simulink model "PC_Quadcopter_Simulation_Alchemist"  (R2023b)
settings: Solver=ode4  StartTime=0  StopTime=Tf  FixedStep=Ts  MaxStep=0.06  RelTol=1e-3  EnableMultiTasking=on
model workspace (MAT data in the model file):
  Sig : Simulink.Signal (value not decoded)
values from neighbouring files (symbols this model uses):
  den_Pphi = conv(den_Qphi, num_Gphi)    [PC_Quadcopter_Alchemist_woDOBC.m]    (also in workingOcto.m)
  den_Ppsi = conv(den_Qpsi, num_Gpsi)    [PC_Quadcopter_Alchemist_woDOBC.m]    (also in workingOcto.m)
  den_Ptheta = conv(den_Qtheta, num_Gtheta)    [PC_Quadcopter_Alchemist_woDOBC.m]    (also in workingOcto.m)
  den_Px = conv(den_Qx, num_Gx)    [PC_Quadcopter_Alchemist_woDOBC.m]    (also in workingOcto.m)
  den_Py = conv(den_Qy, num_Gy)    [PC_Quadcopter_Alchemist_woDOBC.m]    (also in workingOcto.m)
  den_Pz = conv(den_Qz, num_Gz)    [PC_Quadcopter_Alchemist_woDOBC.m]    (also in workingOcto.m)
  Dist_Amp_phi = 0    [PC_Quadcopter_Alchemist_woDOBC.m]    (also in workingOcto.m)
  Dist_Amp_psi = 0    [PC_Quadcopter_Alchemist_woDOBC.m]    (also in workingOcto.m)
  Dist_Amp_theta = 0    [PC_Quadcopter_Alchemist_woDOBC.m]    (also in workingOcto.m)
  Dist_Amp_x = 0    [PC_Quadcopter_Alchemist_woDOBC.m]    (also in workingOcto.m)
  Dist_Amp_y = 0    [PC_Quadcopter_Alchemist_woDOBC.m]    (also in workingOcto.m)
  Dist_Amp_z = 0    [PC_Quadcopter_Alchemist_woDOBC.m]    (also in workingOcto.m)
  Dist_Freq_phi = 0    [PC_Quadcopter_Alchemist_woDOBC.m]    (also in workingOcto.m)
  Dist_Freq_psi = 0    [PC_Quadcopter_Alchemist_woDOBC.m]    (also in workingOcto.m)
  Dist_Freq_theta = 0    [PC_Quadcopter_Alchemist_woDOBC.m]    (also in workingOcto.m)
  Dist_Freq_x = 0    [PC_Quadcopter_Alchemist_woDOBC.m]    (also in workingOcto.m)
  Dist_Freq_y = 0    [PC_Quadcopter_Alchemist_woDOBC.m]    (also in workingOcto.m)
  Dist_Freq_z = 0    [PC_Quadcopter_Alchemist_woDOBC.m]    (also in workingOcto.m)
  Dist_mean_phi = 0    [PC_Quadcopter_Alchemist_woDOBC.m]    (also in workingOcto.m)
  Dist_mean_psi = 0    [PC_Quadcopter_Alchemist_woDOBC.m]    (also in workingOcto.m)
  Dist_mean_theta = 0    [PC_Quadcopter_Alchemist_woDOBC.m]    (also in workingOcto.m)
  Dist_mean_x = 0    [PC_Quadcopter_Alchemist_woDOBC.m]    (also in workingOcto.m)
  Dist_mean_y = 0    [PC_Quadcopter_Alchemist_woDOBC.m]    (also in workingOcto.m)
  Dist_mean_z = 0    [PC_Quadcopter_Alchemist_woDOBC.m]    (also in workingOcto.m)
  Dist_Var_phi = 0    [PC_Quadcopter_Alchemist_woDOBC.m]    (also in workingOcto.m)
  Dist_Var_psi = 0    [PC_Quadcopter_Alchemist_woDOBC.m]    (also in workingOcto.m)
  Dist_Var_theta = 0    [PC_Quadcopter_Alchemist_woDOBC.m]    (also in workingOcto.m)
  Dist_Var_x = 0    [PC_Quadcopter_Alchemist_woDOBC.m]    (also in workingOcto.m)
  Dist_Var_y = 0    [PC_Quadcopter_Alchemist_woDOBC.m]    (also in workingOcto.m)
  Dist_Var_z = 0    [PC_Quadcopter_Alchemist_woDOBC.m]    (also in workingOcto.m)
  DISTURBANCE = 0    [PC_Quadcopter_Alchemist_woDOBC.m]    (also in workingOcto.m)
  DOBC_phi = 0    [PC_Quadcopter_Alchemist_woDOBC.m]    (also in workingOcto.m)
  DOBC_psi = 0    [PC_Quadcopter_Alchemist_woDOBC.m]    (also in workingOcto.m)
  DOBC_theta = 0    [PC_Quadcopter_Alchemist_woDOBC.m]    (also in workingOcto.m)
  DOBC_x = 0    [PC_Quadcopter_Alchemist_woDOBC.m]    (also in workingOcto.m)
  DOBC_y = 0    [PC_Quadcopter_Alchemist_woDOBC.m]    (also in workingOcto.m)
  DOBC_z = 0    [PC_Quadcopter_Alchemist_woDOBC.m]    (also in workingOcto.m)
  GO = (sqrt((m*g)/(8*ct))-b)/cr    [PC_Quadcopter_Alchemist_woDOBC.m]    (also in workingOcto.m)
  IC =     [Hover_1m.mat]    (also in quadcopterDynamicsSFunction_Alchemist.m = block.DialogPrm(2).Data)
  INPUT_MODE_PHI = 0    [PC_Quadcopter_Alchemist_woDOBC.m]    (also in workingOcto.m)
  INPUT_MODE_THETA = 0    [PC_Quadcopter_Alchemist_woDOBC.m]    (also in workingOcto.m)
  INPUT_MODE_U = 0    [PC_Quadcopter_Alchemist_woDOBC.m]    (also in workingOcto.m)
  INPUT_MODE_V = 0    [PC_Quadcopter_Alchemist_woDOBC.m]    (also in workingOcto.m)
  Kd_phi = 2*Zc_phi*Wc_phi*Jx/Kphi    [PC_Quadcopter_Alchemist_woDOBC.m]    (also in workingOcto.m)
  Kd_psi = 2*Zc_psi*Wc_psi*Jz/Kpsi    [PC_Quadcopter_Alchemist_woDOBC.m]    (also in workingOcto.m)
  Kd_theta = 2*Zc_theta*Wc_theta*Jy/Ktheta    [PC_Quadcopter_Alchemist_woDOBC.m]    (also in workingOcto.m)
  Kd_u = Kp_u/50    [PC_Quadcopter_Alchemist_woDOBC.m]    (also in workingOcto.m)
  Kd_v = Kp_v/70    [PC_Quadcopter_Alchemist_woDOBC.m]    (also in workingOcto.m)
  Kd_x = Kp_x/5    (= 0.0710753921948)    [PC_Quadcopter_Alchemist_woDOBC.m]    (also in workingOcto.m = Kp_x/5)
  Kd_y = Kp_y/5    (= 0.014215078439)    [PC_Quadcopter_Alchemist_woDOBC.m]    (also in workingOcto.m = Kp_y/5)
  Kd_z = 2*Zc_z*Wc_z*m/Kz    [PC_Quadcopter_Alchemist_woDOBC.m]    (also in workingOcto.m = Kp_z/10)
  Ki_phi = Kp_phi/10    [PC_Quadcopter_Alchemist_woDOBC.m]    (also in workingOcto.m)
  Ki_psi = Kp_psi/20    [PC_Quadcopter_Alchemist_woDOBC.m]    (also in workingOcto.m)
  Ki_theta = Kp_theta/10    [PC_Quadcopter_Alchemist_woDOBC.m]    (also in workingOcto.m)
  Ki_u = Wc_u^2/g * 0.7    [PC_Quadcopter_Alchemist_woDOBC.m]    (also in workingOcto.m)
  Ki_v = Wc_v^2/g * 0.7    [PC_Quadcopter_Alchemist_woDOBC.m]    (also in workingOcto.m)
  Ki_x = Wc_x^2 * 0.7    (= 0.0442158277169)    [PC_Quadcopter_Alchemist_woDOBC.m]    (also in workingOcto.m = Wc_x^2 * 0.7)
  Ki_y = Wc_y^2 * 0.7    (= 0.00176863310868)    [PC_Quadcopter_Alchemist_woDOBC.m]    (also in workingOcto.m = Wc_y^2 * 0.7)
  Ki_z = 0    [PC_Quadcopter_Alchemist_woDOBC.m]    (also in workingOcto.m = Wc_z^2)
  Kp_phi = Wc_phi^2*Jx/Kphi    [PC_Quadcopter_Alchemist_woDOBC.m]    (also in workingOcto.m)
  Kp_psi = Wc_psi^2*Jz/Kpsi    [PC_Quadcopter_Alchemist_woDOBC.m]    (also in workingOcto.m)
  Kp_theta = Wc_theta^2*Jy/Ktheta    [PC_Quadcopter_Alchemist_woDOBC.m]    (also in workingOcto.m)
  Kp_u = 2*Zc_u*Wc_u/g    [PC_Quadcopter_Alchemist_woDOBC.m]    (also in workingOcto.m)
  Kp_v = 2*Zc_v*Wc_v/g    [PC_Quadcopter_Alchemist_woDOBC.m]    (also in workingOcto.m)
  Kp_x = 2*Wc_x*Zc_x    (= 0.355376960974)    [PC_Quadcopter_Alchemist_woDOBC.m]    (also in workingOcto.m = 2*Wc_x*Zc_x)
  Kp_y = 2*Wc_y*Zc_y    (= 0.0710753921948)    [PC_Quadcopter_Alchemist_woDOBC.m]    (also in workingOcto.m = 2*Wc_y*Zc_y)
  Kp_z = Wc_z^2*Jz/Kz    [PC_Quadcopter_Alchemist_woDOBC.m]    (also in workingOcto.m = 2*Wc_z*Zc_z)
  NOISE = 0    [PC_Quadcopter_Alchemist_woDOBC.m]    (also in workingOcto.m)
  num_Pphi = conv(num_Qphi, den_Gphi)    [PC_Quadcopter_Alchemist_woDOBC.m]    (also in workingOcto.m)
  num_Ppsi = conv(num_Qpsi, den_Gpsi)    [PC_Quadcopter_Alchemist_woDOBC.m]    (also in workingOcto.m)
  num_Ptheta = conv(num_Qtheta, den_Gtheta)    [PC_Quadcopter_Alchemist_woDOBC.m]    (also in workingOcto.m)
  num_Px = conv(num_Qx, den_Gx)    [PC_Quadcopter_Alchemist_woDOBC.m]    (also in workingOcto.m)
  num_Py = conv(num_Qy, den_Gy)    [PC_Quadcopter_Alchemist_woDOBC.m]    (also in workingOcto.m)
  num_Pz = conv(num_Qz, den_Gz)    [PC_Quadcopter_Alchemist_woDOBC.m]    (also in workingOcto.m)
  Phid = deg2rad(1)    [PC_Quadcopter_Alchemist_woDOBC.m]    (also in workingOcto.m = deg2rad(5))
  start_time = 5    [PC_Quadcopter_Alchemist_woDOBC.m]    (also in workingOcto.m = 1)
  step_0_ramp_1 = 0    [PC_Quadcopter_Alchemist_woDOBC.m]    (also in workingOcto.m)
  Thetad = deg2rad(1)    [PC_Quadcopter_Alchemist_woDOBC.m]    (also in workingOcto.m = deg2rad(0))
  Ts = 0.01    [PC_Quadcopter_Alchemist_woDOBC.m]    (also in workingOcto.m)
  Ud = 0    [PC_Quadcopter_Alchemist_woDOBC.m]    (also in workingOcto.m)
  Var_phi = 0.005^2    (= 2.5e-05)    [PC_Quadcopter_Alchemist_woDOBC.m]    (also in workingOcto.m)
  Var_psi = 0.005^2    (= 2.5e-05)    [PC_Quadcopter_Alchemist_woDOBC.m]    (also in workingOcto.m)
  Var_theta = 0.005^2    (= 2.5e-05)    [PC_Quadcopter_Alchemist_woDOBC.m]    (also in workingOcto.m)
  Var_u = 0.01^2    (= 0.0001)    [PC_Quadcopter_Alchemist_woDOBC.m]    (also in workingOcto.m)
  Var_v = 0.01^2    (= 0.0001)    [PC_Quadcopter_Alchemist_woDOBC.m]    (also in workingOcto.m)
  Var_w = 0.01^2    (= 0.0001)    [PC_Quadcopter_Alchemist_woDOBC.m]    (also in workingOcto.m)
  Var_x = 0.01^2    (= 0.0001)    [PC_Quadcopter_Alchemist_woDOBC.m]    (also in workingOcto.m)
  Var_y = 0.01^2    (= 0.0001)    [PC_Quadcopter_Alchemist_woDOBC.m]    (also in workingOcto.m)
  Var_z = 0.01^2    (= 0.0001)    [PC_Quadcopter_Alchemist_woDOBC.m]    (also in workingOcto.m)
  Vd = 0    [PC_Quadcopter_Alchemist_woDOBC.m]    (also in workingOcto.m)
  Vz = 0.1    [PC_Quadcopter_Alchemist_woDOBC.m]    (also in workingOcto.m)
  Xd = 0    [PC_Quadcopter_Alchemist_woDOBC.m]    (also in workingOcto.m = 1)
  Yd = 0    [PC_Quadcopter_Alchemist_woDOBC.m]    (also in workingOcto.m = 1)
  Zd = 2    [PC_Quadcopter_Alchemist_woDOBC.m]    (also in workingOcto.m = 1)
undefined symbols (not defined in the file or in its folder): den_Qphi, den_Qpsi, den_Qtheta, den_Qx, den_Qy, den_Qz, num_Qphi, num_Qpsi, num_Qtheta, num_Qx, num_Qy, num_Qz, quadModel
libraries: simulink x10, slpidlib x2, sharedtransform x1, uavutilslib x1
(part 2 of 2)

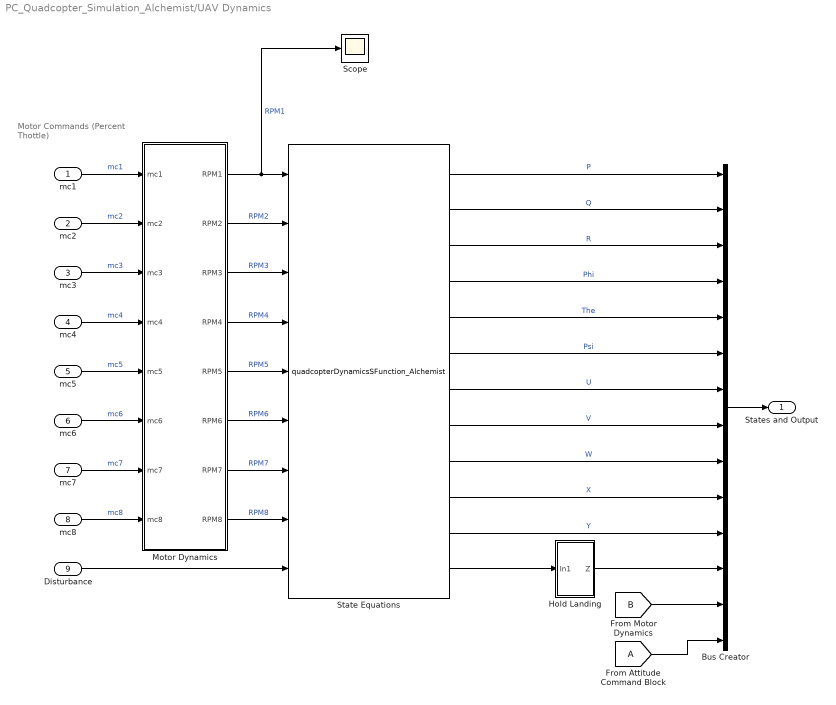
== system PC_Quadcopter_Simulation_Alchemist/UAV Dynamics ==
  note: Motor Commands
      | (Percent Thottle)
  mc1 : Inport
  mc2 : Inport  Port=2
  mc3 : Inport  Port=3
  mc4 : Inport  Port=4
  mc5 : Inport  Port=5
  mc6 : Inport  Port=6
  mc7 : Inport  Port=7
  mc8 : Inport  Port=8
  Disturbance : Inport  Port=9
  Bus Creator : BusCreator  Inputs='P','Q','R','Phi','The','Psi','U','V','W','X','Y','Z','mc and RPM','Attitude_Cmd'
  From Attitude Command Block : From  TagVisibility=global
  Hold Landing : Subsystem
  Motor Dynamics : Subsystem
  Scope : Scope
  State Equations : M-S-Function  FunctionName=quadcopterDynamicsSFunction_Alchemist  Parameters=quadModel, IC
      mask Display:
      | port_label('input', 1, 'RPM1')
      | port_label('input', 2, 'RPM2')
      | port_label('input', 3, 'RPM3')
      | port_label('input', 4, 'RPM4')
      | port_label('input', 5, 'Disturbances')
      | port_label('output', 1, 'P')
      | port_label('output', 2, 'Q')
      | port_label('output', 3, 'R')
      | port_label('output', 4, 'Phi')
      | port_label('output', 5, 'The')
      | port_label('output', 6, 'Psi')
      | port_label('output', 7, 'U')
      | port_label('output', 8, 'V')
      | port_label('output', 9, 'W')
      | port_label('output', 10, 'X')
      | port_label('output', 11, 'Y')
      | port_label('output', 12, 'Z')
  States and Output : Outport  VectorParamsAs1DForOutWhenUnconnected=off
  wires:
  [B] -> Bus Creator/13
  From Attitude Command Block/1 -> Bus Creator/14
  mc2/1 -> Motor Dynamics/2(mc2)  "mc2"
  mc3/1 -> Motor Dynamics/3(mc3)  "mc3"
  mc4/1 -> Motor Dynamics/4(mc4)  "mc4"
  mc1/1 -> Motor Dynamics/1(mc1)  "mc1"
  Motor Dynamics/3(RPM3) -> State Equations/3  "RPM3"
  Motor Dynamics/2(RPM2) -> State Equations/2  "RPM2"
  Bus Creator/1 -> States and Output/1
  State Equations/11 -> Bus Creator/11  "Y"
  State Equations/10 -> Bus Creator/10  "X"
  State Equations/9 -> Bus Creator/9  "W"
  State Equations/8 -> Bus Creator/8  "V"
  State Equations/7 -> Bus Creator/7  "U"
  State Equations/6 -> Bus Creator/6  "Psi"
  State Equations/5 -> Bus Creator/5  "The"
  State Equations/4 -> Bus Creator/4  "Phi"
  State Equations/3 -> Bus Creator/3  "R"
  State Equations/2 -> Bus Creator/2  "Q"
  State Equations/1 -> Bus Creator/1  "P"
  Motor Dynamics/1(RPM1) -> Scope/1, State Equations/1  "RPM1"
  mc5/1 -> Motor Dynamics/5(mc5)  "mc5"
  mc6/1 -> Motor Dynamics/6(mc6)  "mc6"
  State Equations/12 -> Hold Landing/1(In1)
  Hold Landing/1(Z) -> Bus Creator/12
  mc7/1 -> Motor Dynamics/7(mc7)  "mc7"
  mc8/1 -> Motor Dynamics/8(mc8)  "mc8"
  Disturbance/1 -> State Equations/9
  Motor Dynamics/4(RPM4) -> State Equations/4  "RPM4"
  Motor Dynamics/5(RPM5) -> State Equations/5  "RPM5"
  Motor Dynamics/6(RPM6) -> State Equations/6  "RPM6"
  Motor Dynamics/7(RPM7) -> State Equations/7  "RPM7"
  Motor Dynamics/8(RPM8) -> State Equations/8  "RPM8"

== system PC_Quadcopter_Simulation_Alchemist/Attitude & Altitude Controller/Altitude (Z) Control ==
  note: ez
  note: Improve to use rotation matrix and euler angles...
      | maybe with saturation?
  Desired Z : Inport
  Z State : Inport  Port=2
  Bus Selector : BusSelector  OutputSignals=Alt_cmd
  Derivative : Derivative
  Gravity Offset (Level Flight) : Constant  Value=GOffset
  Integrator Limited : Integrator  LimitOutput=on  UpperSaturationLimit=USat  LowerSaturationLimit=LSat
  Kdz : Gain  Gain=Kdz
  Kiz : Gain  Gain=Kiz
  Kpz : Gain  Gain=Kpz
  Sum : Sum  Inputs=|+-
  Sum2 : Sum  Inputs=+++-
  Alt. (Z) Correction : Outport  VectorParamsAs1DForOutWhenUnconnected=off
  wires:
  Derivative/1 -> Kdz/1
  Bus Selector/1 -> Sum/1  "<Alt_cmd>"
  Integrator Limited/1 -> Kiz/1
  Kdz/1 -> Sum2/4  "D Corr"
  Kiz/1 -> Sum2/3  "I Corr"
  Sum/1 -> Kpz/1, Integrator Limited/1  "Error"
  Kpz/1 -> Sum2/2  "P Corr"
  Sum2/1 -> Alt. (Z) Correction/1
  Z State/1 -> Sum/2, Derivative/1
  Desired Z/1 -> Bus Selector/1
  Gravity Offset (Level Flight)/1 -> Sum2/1

== system PC_Quadcopter_Simulation_Alchemist/Attitude & Altitude Controller/DOBC_Phi ==
  In2 : Inport
  Phi : Inport  Port=2
  Gain3 : Gain  Gain=DOBC_phi
  Q(s)*inv(G(s))3 : TransferFcn  Numerator=num_Pphi  Denominator=den_Pphi
  Q(s)3 : TransferFcn  Numerator=num_Qphi  Denominator=den_Qphi
  Sum6 : Sum  Inputs=|+-
  Sum9 : Sum  Inputs=+|-
  Roll (Phi) Correction : Outport
  wires:
  Sum9/1 -> Gain3/1
  Q(s)3/1 -> Sum9/2
  Sum6/1 -> Roll (Phi) Correction/1, Q(s)3/1
  In2/1 -> Sum6/1
  Q(s)*inv(G(s))3/1 -> Sum9/1
  Gain3/1 -> Sum6/2
  Phi/1 -> Q(s)*inv(G(s))3/1

== system PC_Quadcopter_Simulation_Alchemist/Attitude & Altitude Controller/DOBC_Psi ==
  In2 : Inport
  Psi : Inport  Port=2
  Gain1 : Gain  Gain=DOBC_psi
  Q(s)*inv(G(s))1 : TransferFcn  Numerator=num_Ppsi  Denominator=den_Ppsi
  Q(s)1 : TransferFcn  Numerator=num_Qpsi  Denominator=den_Qpsi
  Sum4 : Sum  Inputs=|+-
  Sum7 : Sum  Inputs=+|-
  Yaw (Psi) Correction : Outport
  wires:
  Sum7/1 -> Gain1/1
  Psi/1 -> Q(s)*inv(G(s))1/1
  Sum4/1 -> Yaw (Psi) Correction/1, Q(s)1/1
  Q(s)1/1 -> Sum7/2
  Q(s)*inv(G(s))1/1 -> Sum7/1
  Gain1/1 -> Sum4/2
  In2/1 -> Sum4/1

== system PC_Quadcopter_Simulation_Alchemist/Attitude & Altitude Controller/DOBC_Theta ==
  In2 : Inport
  Theta : Inport  Port=2
  Gain2 : Gain  Gain=DOBC_theta
  Q(s)*inv(G(s))2 : TransferFcn  Numerator=num_Ptheta  Denominator=den_Ptheta
  Q(s)2 : TransferFcn  Numerator=num_Qtheta  Denominator=den_Qtheta
  Sum5 : Sum  Inputs=|+-
  Sum8 : Sum  Inputs=+|-
  Pitch (Theta) Correction : Outport
  wires:
  Gain2/1 -> Sum5/2
  Sum5/1 -> Pitch (Theta) Correction/1, Q(s)2/1
  Sum8/1 -> Gain2/1
  Q(s)*inv(G(s))2/1 -> Sum8/1
  In2/1 -> Sum5/1
  Q(s)2/1 -> Sum8/2
  Theta/1 -> Q(s)*inv(G(s))2/1

== system PC_Quadcopter_Simulation_Alchemist/Attitude & Altitude Controller/DOBC_Z ==
  In1 : Inport
  Z : Inport  Port=2
  Gain : Gain  Gain=DOBC_z
  Q(s) : TransferFcn  Numerator=num_Qz  Denominator=den_Qz
  Q(s)*inv(G(s)) : TransferFcn  Numerator=num_Pz  Denominator=den_Pz
  Sum : Sum  Inputs=+|-
  Sum1 : Sum  Inputs=|+-
  Out1 : Outport
  wires:
  Sum/1 -> Gain/1
  Sum1/1 -> Out1/1, Q(s)/1
  In1/1 -> Sum1/1
  Gain/1 -> Sum1/2
  Q(s)*inv(G(s))/1 -> Sum/1
  Q(s)/1 -> Sum/2
  Z/1 -> Q(s)*inv(G(s))/1

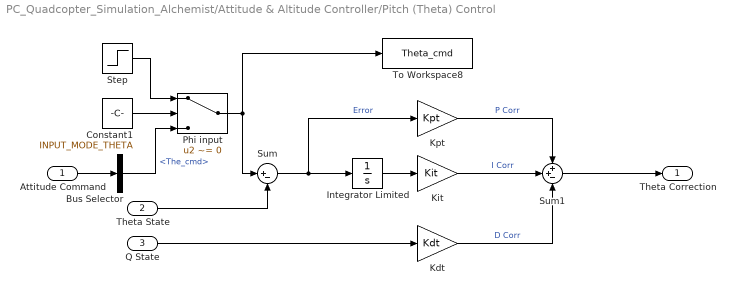
== system PC_Quadcopter_Simulation_Alchemist/Attitude & Altitude Controller/Pitch (Theta) Control ==
  Attitude Command : Inport
  Theta State : Inport  Port=2
  Q State : Inport  Port=3
  Bus Selector : BusSelector  OutputSignals=The_cmd
  Constant1 : Constant  Value=INPUT_MODE_THETA
  Integrator Limited : Integrator  LimitOutput=on  UpperSaturationLimit=USat  LowerSaturationLimit=LSat
  Kdt : Gain  Gain=Kdt
  Kit : Gain  Gain=Kit
  Kpt : Gain  Gain=Kpt
  Phi input : Switch  Criteria=u2 ~= 0  SaturateOnIntegerOverflow=off  InputSameDT=off
  Step : Step  Time=start_time  After=Thetad  SampleTime=0
  Sum : Sum  Inputs=|+-
  Sum1 : Sum  Inputs=++-
  To Workspace8 : ToWorkspace  VariableName=Theta_cmd  SampleTime=-1
      settings: Save2DSignal=2-D array (concatenate along first dimension)
  Theta Correction : Outport  VectorParamsAs1DForOutWhenUnconnected=off
  wires:
  Q State/1 -> Kdt/1
  Bus Selector/1 -> Phi input/3  "<The_cmd>"
  Integrator Limited/1 -> Kit/1
  Kit/1 -> Sum1/2  "I Corr"
  Kdt/1 -> Sum1/3  "D Corr"
  Kpt/1 -> Sum1/1  "P Corr"
  Sum1/1 -> Theta Correction/1
  Theta State/1 -> Sum/2
  Attitude Command/1 -> Bus Selector/1
  Sum/1 -> Kpt/1, Integrator Limited/1  "Error"
  Phi input/1 -> Sum/1, To Workspace8/1
  Step/1 -> Phi input/1
  Constant1/1 -> Phi input/2

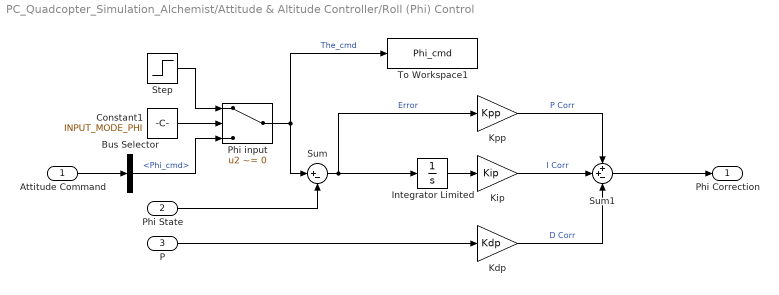
== system PC_Quadcopter_Simulation_Alchemist/Attitude & Altitude Controller/Roll (Phi) Control  ==
  "Attitude Command " : Inport
  Phi State : Inport  Port=2
  P : Inport  Port=3
  Bus Selector : BusSelector  OutputSignals=Phi_cmd
  Constant1 : Constant  Value=INPUT_MODE_PHI
  Integrator Limited : Integrator  LimitOutput=on  UpperSaturationLimit=USat  LowerSaturationLimit=LSat
  Kdp : Gain  Gain=Kdp
  Kip : Gain  Gain=Kip
  Kpp : Gain  Gain=Kpp
  Phi input : Switch  Criteria=u2 ~= 0  SaturateOnIntegerOverflow=off  InputSameDT=off
  Step : Step  Time=start_time  After=Phid  SampleTime=0
  Sum : Sum  Inputs=|+-
  Sum1 : Sum  Inputs=++-
  To Workspace1 : ToWorkspace  VariableName=Phi_cmd  SampleTime=-1
      settings: Save2DSignal=2-D array (concatenate along first dimension)
  Phi Correction : Outport  VectorParamsAs1DForOutWhenUnconnected=off
  wires:
  P/1 -> Kdp/1
  Bus Selector/1 -> Phi input/3  "<Phi_cmd>"
  "Attitude Command "/1 -> Bus Selector/1
  Integrator Limited/1 -> Kip/1
  Kip/1 -> Sum1/2  "I Corr"
  Kdp/1 -> Sum1/3  "D Corr"
  Kpp/1 -> Sum1/1  "P Corr"
  Sum1/1 -> Phi Correction/1
  Phi State/1 -> Sum/2
  Sum/1 -> Kpp/1, Integrator Limited/1  "Error"
  Step/1 -> Phi input/1
  Constant1/1 -> Phi input/2
  Phi input/1 -> To Workspace1/1, Sum/1  "The_cmd"

== system PC_Quadcopter_Simulation_Alchemist/Attitude & Altitude Controller/Yaw (Psi) Control ==
  Attitude Command : Inport
  Psi State : Inport  Port=2
  R State : Inport  Port=3
  Bus Selector : BusSelector  OutputSignals=Psi_cmd
  Integrator Limited : Integrator  LimitOutput=on  UpperSaturationLimit=USat  LowerSaturationLimit=LSat
  Kds : Gain  Gain=Kds
  Kit : Gain  Gain=Kis
  Kps : Gain  Gain=Kps
  Sum : Sum  Inputs=|+-
  Sum1 : Sum  Inputs=++-
  To Workspace3 : ToWorkspace  VariableName=Psi_cmd  SampleTime=-1
      settings: Save2DSignal=2-D array (concatenate along first dimension)
  Psi Correction : Outport  VectorParamsAs1DForOutWhenUnconnected=off
  wires:
  R State/1 -> Kds/1
  Bus Selector/1 -> To Workspace3/1, Sum/1  "<Psi_cmd>"
  Integrator Limited/1 -> Kit/1
  Kit/1 -> Sum1/2  "I Corr"
  Kds/1 -> Sum1/3  "D Corr"
  Kps/1 -> Sum1/1  "P Corr"
  Psi State/1 -> Sum/2
  Sum1/1 -> Psi Correction/1
  Attitude Command/1 -> Bus Selector/1
  Sum/1 -> Kps/1, Integrator Limited/1  "Error"

== system PC_Quadcopter_Simulation_Alchemist/Position and Velocity Controller/DOBC_X ==
  In1 : Inport
  X : Inport  Port=2
  Gain : Gain  Gain=DOBC_x
  Q(s) : TransferFcn  Numerator=num_Qx  Denominator=den_Qx
  Q(s)*inv(G(s)) : TransferFcn  Numerator=num_Px  Denominator=den_Px
  Sum : Sum  Inputs=+|-
  Sum1 : Sum  Inputs=|+-
  Out1 : Outport
  wires:
  Sum/1 -> Gain/1
  Sum1/1 -> Out1/1, Q(s)/1
  In1/1 -> Sum1/1
  Gain/1 -> Sum1/2
  Q(s)*inv(G(s))/1 -> Sum/1
  Q(s)/1 -> Sum/2
  X/1 -> Q(s)*inv(G(s))/1

== system PC_Quadcopter_Simulation_Alchemist/Position and Velocity Controller/DOBC_Y ==
  In1 : Inport
  Y : Inport  Port=2
  Gain : Gain  Gain=DOBC_y
  Q(s) : TransferFcn  Numerator=num_Qy  Denominator=den_Qy
  Q(s)*inv(G(s)) : TransferFcn  Numerator=num_Py  Denominator=den_Py
  Sum : Sum  Inputs=+|-
  Sum1 : Sum  Inputs=|+-
  Out1 : Outport
  wires:
  Y/1 -> Q(s)*inv(G(s))/1
  Q(s)/1 -> Sum/2
  Q(s)*inv(G(s))/1 -> Sum/1
  Gain/1 -> Sum1/2
  In1/1 -> Sum1/1
  Sum1/1 -> Q(s)/1, Out1/1
  Sum/1 -> Gain/1

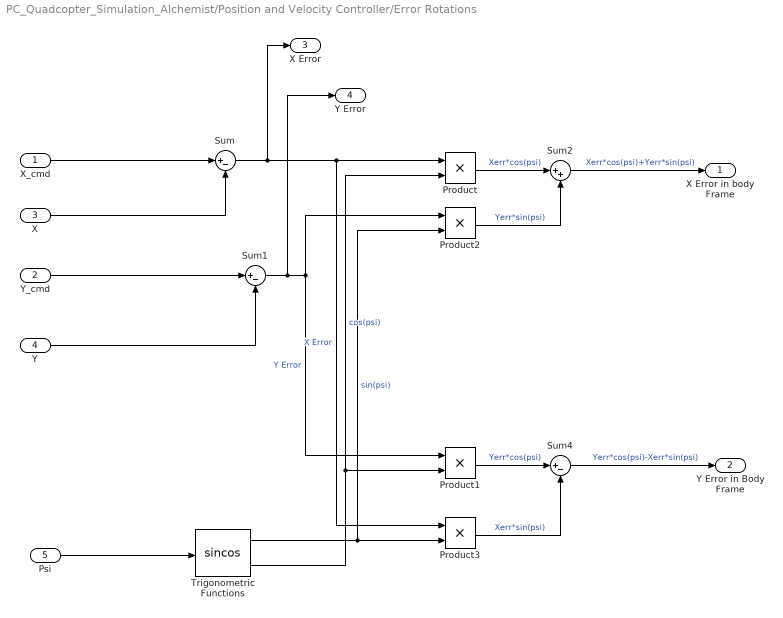
== system PC_Quadcopter_Simulation_Alchemist/Position and Velocity Controller/Error Rotations ==
  X_cmd : Inport
  Y_cmd : Inport  Port=2
  X : Inport  Port=3
  Y : Inport  Port=4
  Psi : Inport  Port=5
  Product{,1..3} (4 alike) : Product
  Sum : Sum  Inputs=|+-
  Sum1 : Sum  Inputs=|+-
  Sum2 : Sum  Inputs=|++
  Sum4 : Sum  Inputs=|+-
  Trigonometric Functions : Trigonometry  Operator=sincos
  X Error in body Frame : Outport
  Y Error in Body Frame : Outport  Port=2
  X Error : Outport  Port=3
  Y Error : Outport  Port=4
  wires:
  Sum4/1 -> Y Error in Body Frame/1  "Yerr*cos(psi)-Xerr*sin(psi)"
  Product3/1 -> Sum4/2  "Xerr*sin(psi)"
  Sum1/1 -> Y Error/1, Product2/1, Product1/1  "Y Error"
  Trigonometric Functions/1 -> Product2/2, Product3/2  "sin(psi)"
  Sum2/1 -> X Error in body Frame/1  "Xerr*cos(psi)+Yerr*sin(psi)"
  Y_cmd/1 -> Sum1/1
  X_cmd/1 -> Sum/1
  X/1 -> Sum/2
  Y/1 -> Sum1/2
  Sum/1 -> X Error/1, Product3/1, Product/1  "X Error"
  Trigonometric Functions/2 -> Product/2, Product1/2  "cos(psi)"
  Product/1 -> Sum2/1  "Xerr*cos(psi)"
  Product2/1 -> Sum2/2  "Yerr*sin(psi)"
  Product1/1 -> Sum4/1  "Yerr*cos(psi)"
  Psi/1 -> Trigonometric Functions/1

== system PC_Quadcopter_Simulation_Alchemist/Position and Velocity Controller/U Controller ==
  Desired Xb Velocity : Inport
  Xb Velocity : Inport  Port=2
  Attitude Limits_Theta : Saturate  UpperLimit=ASat  LowerLimit=-ASat
  Integrator : Integrator
  Kdt : Gain  Gain=Kd
  Kpt : Gain  Gain=Kp
  Kpt1 : Gain  Gain=Ki_u
  Sum3 : Sum  Inputs=|+-
  Sum6 : Sum  Inputs=++-
  U Derivative : Derivative
  The_cmd : Outport
  wires:
  U Derivative/1 -> Kdt/1
  Attitude Limits_Theta/1 -> The_cmd/1  "The_cmd"
  Sum6/1 -> Attitude Limits_Theta/1
  Sum3/1 -> Integrator/1, Kpt/1  "Velocity Error"
  Xb Velocity/1 -> U Derivative/1, Sum3/2
  Desired Xb Velocity/1 -> Sum3/1
  Integrator/1 -> Kpt1/1
  Kdt/1 -> Sum6/3
  Kpt/1 -> Sum6/2
  Kpt1/1 -> Sum6/1

== system PC_Quadcopter_Simulation_Alchemist/Position and Velocity Controller/V Controller ==
  note: -1 Gain is required because a "negative"
      | angle of Phi induces a positive velocity
      | in the body frame y direction!
  Desired Yb Velocity : Inport
  Yb Velocity : Inport  Port=2
  Attitude Limits_Phi : Saturate  UpperLimit=ASat  LowerLimit=-ASat
  Gain : Gain  Gain=-1
  Integrator : Integrator
  Kdp : Gain  Gain=Kd
  Kpp : Gain  Gain=Kp
  Kpt1 : Gain  Gain=Ki_v
  Sum3 : Sum  Inputs=|+-
  Sum6 : Sum  Inputs=++-
  V Derivative : Derivative
  Phi_cmd : Outport
  wires:
  V Derivative/1 -> Kdp/1
  Attitude Limits_Phi/1 -> Phi_cmd/1  "Phi_cmd"
  Sum6/1 -> Gain/1
  Yb Velocity/1 -> V Derivative/1, Sum3/2
  Desired Yb Velocity/1 -> Sum3/1
  Gain/1 -> Attitude Limits_Phi/1
  Integrator/1 -> Kpt1/1
  Kpt1/1 -> Sum6/1
  Sum3/1 -> Integrator/1, Kpp/1  "Velocity Error"
  Kdp/1 -> Sum6/3
  Kpp/1 -> Sum6/2

== system PC_Quadcopter_Simulation_Alchemist/UAV Dynamics/Hold Landing ==
  In1 : Inport
  Constant : Constant  Value=0
  Delay : Delay  DelayLength=1
  IC : InitialCondition  Value=IC.Z
  Switch : Switch  Criteria=u2 > Threshold  SaturateOnIntegerOverflow=off  InputSameDT=off
  Z : Outport
  wires:
  IC/1 -> Switch/2
  Switch/1 -> Z/1, Delay/1  "Z"
  Delay/1 -> IC/1
  Constant/1 -> Switch/3
  In1/1 -> Switch/1

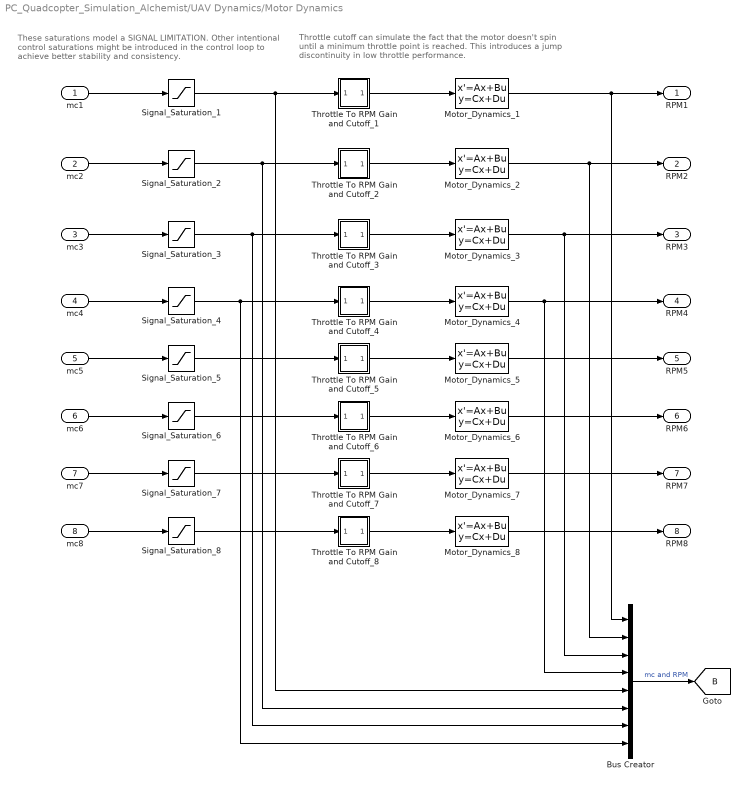
== system PC_Quadcopter_Simulation_Alchemist/UAV Dynamics/Motor Dynamics ==
  note: These saturations model a SIGNAL LIMITATION.
      | Other intentional control saturations might be introduced in the
      | control loop to achieve better stability and consistency.
  note: Throttle cutoff can simulate the fact that the motor doesn't
      | spin until a minimum throttle point is reached. This introduces
      | a jump discontinuity in low throttle performance.
  mc1 : Inport
  mc2 : Inport  Port=2
  mc3 : Inport  Port=3
  mc4 : Inport  Port=4
  mc5 : Inport  Port=5
  mc6 : Inport  Port=6
  mc7 : Inport  Port=7
  mc8 : Inport  Port=8
  Bus Creator : BusCreator  Inputs=8
  Motor_Dynamics_1 : StateSpace  A=-1/quadModel.T  C=1/quadModel.T  D=0  InitialCondition=IC.w1*quadModel.T
  Motor_Dynamics_2 : StateSpace  A=-1/quadModel.T  C=1/quadModel.T  D=0  InitialCondition=IC.w2*quadModel.T
  Motor_Dynamics_3 : StateSpace  A=-1/quadModel.T  C=1/quadModel.T  D=0  InitialCondition=IC.w3*quadModel.T
  Motor_Dynamics_4 : StateSpace  A=-1/quadModel.T  C=1/quadModel.T  D=0  InitialCondition=IC.w4*quadModel.T
  Motor_Dynamics_5 : StateSpace  A=-1/quadModel.T  C=1/quadModel.T  D=0  InitialCondition=IC.w5*quadModel.T
  Motor_Dynamics_6 : StateSpace  A=-1/quadModel.T  C=1/quadModel.T  D=0  InitialCondition=IC.w6*quadModel.T
  Motor_Dynamics_7 : StateSpace  A=-1/quadModel.T  C=1/quadModel.T  D=0  InitialCondition=IC.w7*quadModel.T
  Motor_Dynamics_8 : StateSpace  A=-1/quadModel.T  C=1/quadModel.T  D=0  InitialCondition=IC.w8*quadModel.T
  Signal_Saturation_{1..8} (8 alike) : Saturate  UpperLimit=100  LowerLimit=0
  Throttle To RPM Gain and Cutoff_1 : Subsystem
  Throttle To RPM Gain and Cutoff_2 : Subsystem
  Throttle To RPM Gain and Cutoff_3 : Subsystem
  Throttle To RPM Gain and Cutoff_4 : Subsystem
  Throttle To RPM Gain and Cutoff_5 : Subsystem
  Throttle To RPM Gain and Cutoff_6 : Subsystem
  Throttle To RPM Gain and Cutoff_7 : Subsystem
  Throttle To RPM Gain and Cutoff_8 : Subsystem
  RPM1 : Outport  VectorParamsAs1DForOutWhenUnconnected=off
  RPM2 : Outport  Port=2  VectorParamsAs1DForOutWhenUnconnected=off
  RPM3 : Outport  Port=3  VectorParamsAs1DForOutWhenUnconnected=off
  RPM4 : Outport  Port=4  VectorParamsAs1DForOutWhenUnconnected=off
  RPM5 : Outport  Port=5  VectorParamsAs1DForOutWhenUnconnected=off
  RPM6 : Outport  Port=6  VectorParamsAs1DForOutWhenUnconnected=off
  RPM7 : Outport  Port=7  VectorParamsAs1DForOutWhenUnconnected=off
  RPM8 : Outport  Port=8  VectorParamsAs1DForOutWhenUnconnected=off
  tag scope: B=global
  wires:
  Bus Creator/1 -> [B]  "mc and RPM"
  Motor_Dynamics_4/1 -> RPM4/1, Bus Creator/4
  Motor_Dynamics_3/1 -> RPM3/1, Bus Creator/3
  Motor_Dynamics_2/1 -> RPM2/1, Bus Creator/2
  Motor_Dynamics_1/1 -> RPM1/1, Bus Creator/1
  Throttle To RPM Gain and Cutoff_4/1(Out5) -> Motor_Dynamics_4/1
  Throttle To RPM Gain and Cutoff_3/1(Out5) -> Motor_Dynamics_3/1
  Throttle To RPM Gain and Cutoff_2/1(Out5) -> Motor_Dynamics_2/1
  Throttle To RPM Gain and Cutoff_1/1(Out5) -> Motor_Dynamics_1/1
  Signal_Saturation_4/1 -> Throttle To RPM Gain and Cutoff_4/1(In5), Bus Creator/8
  Signal_Saturation_3/1 -> Throttle To RPM Gain and Cutoff_3/1(In5), Bus Creator/7
  Signal_Saturation_2/1 -> Throttle To RPM Gain and Cutoff_2/1(In5), Bus Creator/6
  Signal_Saturation_1/1 -> Throttle To RPM Gain and Cutoff_1/1(In5), Bus Creator/5
  mc3/1 -> Signal_Saturation_3/1
  mc2/1 -> Signal_Saturation_2/1
  mc4/1 -> Signal_Saturation_4/1
  mc1/1 -> Signal_Saturation_1/1
  mc5/1 -> Signal_Saturation_5/1
  Signal_Saturation_5/1 -> Throttle To RPM Gain and Cutoff_5/1(In5)
  Throttle To RPM Gain and Cutoff_5/1(Out5) -> Motor_Dynamics_5/1
  Motor_Dynamics_5/1 -> RPM5/1
  Motor_Dynamics_6/1 -> RPM6/1
  Throttle To RPM Gain and Cutoff_6/1(Out5) -> Motor_Dynamics_6/1
  Signal_Saturation_6/1 -> Throttle To RPM Gain and Cutoff_6/1(In5)
  mc6/1 -> Signal_Saturation_6/1
  mc7/1 -> Signal_Saturation_7/1
  Signal_Saturation_7/1 -> Throttle To RPM Gain and Cutoff_7/1(In5)
  Throttle To RPM Gain and Cutoff_7/1(Out5) -> Motor_Dynamics_7/1
  Motor_Dynamics_7/1 -> RPM7/1
  mc8/1 -> Signal_Saturation_8/1
  Signal_Saturation_8/1 -> Throttle To RPM Gain and Cutoff_8/1(In5)
  Throttle To RPM Gain and Cutoff_8/1(Out5) -> Motor_Dynamics_8/1
  Motor_Dynamics_8/1 -> RPM8/1

== system PC_Quadcopter_Simulation_Alchemist/UAV Dynamics/Motor Dynamics/Throttle To RPM Gain and Cutoff_1 ==
  note: Output equals linearly scaled RPM
      | for given throttle input if throttle input >=Throttle Cuttoff (minThr)
      | else output is zero.
  In5 : Inport
  Constant : Constant  Value=quadModel.b
  Gain : Gain  Gain=quadModel.cr
  Minimum Throttle Cutoff : simulink/Logic and Bit Operations/Compare To Constant  relop=>=  const=quadModel.minThr  OutDataTypeStr=uint8
  Product : Product
  Sum1 : Sum  Inputs=++|
  Out5 : Outport  VectorParamsAs1DForOutWhenUnconnected=off
  wires:
  Constant/1 -> Sum1/1
  Sum1/1 -> Product/1
  Gain/1 -> Sum1/2
  In5/1 -> Minimum Throttle Cutoff/1, Gain/1
  Product/1 -> Out5/1
  Minimum Throttle Cutoff/1 -> Product/2

== system PC_Quadcopter_Simulation_Alchemist/UAV Dynamics/Motor Dynamics/Throttle To RPM Gain and Cutoff_2 ==
  note: Output equals linearly scaled RPM
      | for given throttle input if throttle input >=Throttle Cuttoff (minThr)
      | else output is zero.
  In5 : Inport
  Constant : Constant  Value=quadModel.b
  Gain : Gain  Gain=quadModel.cr
  Minimum Throttle Cutoff : simulink/Logic and Bit Operations/Compare To Constant  relop=>=  const=quadModel.minThr  OutDataTypeStr=uint8
  Product : Product
  Sum1 : Sum  Inputs=++|
  Out5 : Outport  VectorParamsAs1DForOutWhenUnconnected=off
  wires:
  Constant/1 -> Sum1/1
  Sum1/1 -> Product/1
  Gain/1 -> Sum1/2
  In5/1 -> Minimum Throttle Cutoff/1, Gain/1
  Product/1 -> Out5/1
  Minimum Throttle Cutoff/1 -> Product/2

== system PC_Quadcopter_Simulation_Alchemist/UAV Dynamics/Motor Dynamics/Throttle To RPM Gain and Cutoff_3 ==
  note: Output equals linearly scaled RPM
      | for given throttle input if throttle input >=Throttle Cuttoff (minThr)
      | else output is zero.
  In5 : Inport
  Constant : Constant  Value=quadModel.b
  Gain : Gain  Gain=quadModel.cr
  Minimum Throttle Cutoff : simulink/Logic and Bit Operations/Compare To Constant  relop=>=  const=quadModel.minThr  OutDataTypeStr=uint8
  Product : Product
  Sum1 : Sum  Inputs=++|
  Out5 : Outport  VectorParamsAs1DForOutWhenUnconnected=off
  wires:
  Constant/1 -> Sum1/1
  Sum1/1 -> Product/1
  Gain/1 -> Sum1/2
  In5/1 -> Minimum Throttle Cutoff/1, Gain/1
  Product/1 -> Out5/1
  Minimum Throttle Cutoff/1 -> Product/2

== system PC_Quadcopter_Simulation_Alchemist/UAV Dynamics/Motor Dynamics/Throttle To RPM Gain and Cutoff_4 ==
  note: Output equals linearly scaled RPM
      | for given throttle input if throttle input >=Throttle Cuttoff (minThr)
      | else output is zero.
  In5 : Inport
  Constant : Constant  Value=quadModel.b
  Gain : Gain  Gain=quadModel.cr
  Minimum Throttle Cutoff : simulink/Logic and Bit Operations/Compare To Constant  relop=>=  const=quadModel.minThr  OutDataTypeStr=uint8
  Product : Product
  Sum1 : Sum  Inputs=++|
  Out5 : Outport  VectorParamsAs1DForOutWhenUnconnected=off
  wires:
  Constant/1 -> Sum1/1
  Sum1/1 -> Product/1
  Gain/1 -> Sum1/2
  In5/1 -> Minimum Throttle Cutoff/1, Gain/1
  Product/1 -> Out5/1
  Minimum Throttle Cutoff/1 -> Product/2

== system PC_Quadcopter_Simulation_Alchemist/UAV Dynamics/Motor Dynamics/Throttle To RPM Gain and Cutoff_5 ==
  note: Output equals linearly scaled RPM
      | for given throttle input if throttle input >=Throttle Cuttoff (minThr)
      | else output is zero.
  In5 : Inport
  Constant : Constant  Value=quadModel.b
  Gain : Gain  Gain=quadModel.cr
  Minimum Throttle Cutoff : simulink/Logic and Bit Operations/Compare To Constant  relop=>=  const=quadModel.minThr  OutDataTypeStr=uint8
  Product : Product
  Sum1 : Sum  Inputs=++|
  Out5 : Outport  VectorParamsAs1DForOutWhenUnconnected=off
  wires:
  Minimum Throttle Cutoff/1 -> Product/2
  Product/1 -> Out5/1
  In5/1 -> Gain/1, Minimum Throttle Cutoff/1
  Gain/1 -> Sum1/2
  Sum1/1 -> Product/1
  Constant/1 -> Sum1/1

== system PC_Quadcopter_Simulation_Alchemist/UAV Dynamics/Motor Dynamics/Throttle To RPM Gain and Cutoff_6 ==
  note: Output equals linearly scaled RPM
      | for given throttle input if throttle input >=Throttle Cuttoff (minThr)
      | else output is zero.
  In5 : Inport
  Constant : Constant  Value=quadModel.b
  Gain : Gain  Gain=quadModel.cr
  Minimum Throttle Cutoff : simulink/Logic and Bit Operations/Compare To Constant  relop=>=  const=quadModel.minThr  OutDataTypeStr=uint8
  Product : Product
  Sum1 : Sum  Inputs=++|
  Out5 : Outport  VectorParamsAs1DForOutWhenUnconnected=off
  wires:
  Constant/1 -> Sum1/1
  Sum1/1 -> Product/1
  Gain/1 -> Sum1/2
  In5/1 -> Minimum Throttle Cutoff/1, Gain/1
  Product/1 -> Out5/1
  Minimum Throttle Cutoff/1 -> Product/2

== system PC_Quadcopter_Simulation_Alchemist/UAV Dynamics/Motor Dynamics/Throttle To RPM Gain and Cutoff_7 ==
  note: Output equals linearly scaled RPM
      | for given throttle input if throttle input >=Throttle Cuttoff (minThr)
      | else output is zero.
  In5 : Inport
  Constant : Constant  Value=quadModel.b
  Gain : Gain  Gain=quadModel.cr
  Minimum Throttle Cutoff : simulink/Logic and Bit Operations/Compare To Constant  relop=>=  const=quadModel.minThr  OutDataTypeStr=uint8
  Product : Product
  Sum1 : Sum  Inputs=++|
  Out5 : Outport  VectorParamsAs1DForOutWhenUnconnected=off
  wires:
  Constant/1 -> Sum1/1
  Sum1/1 -> Product/1
  Gain/1 -> Sum1/2
  In5/1 -> Minimum Throttle Cutoff/1, Gain/1
  Product/1 -> Out5/1
  Minimum Throttle Cutoff/1 -> Product/2

== system PC_Quadcopter_Simulation_Alchemist/UAV Dynamics/Motor Dynamics/Throttle To RPM Gain and Cutoff_8 ==
  note: Output equals linearly scaled RPM
      | for given throttle input if throttle input >=Throttle Cuttoff (minThr)
      | else output is zero.
  In5 : Inport
  Constant : Constant  Value=quadModel.b
  Gain : Gain  Gain=quadModel.cr
  Minimum Throttle Cutoff : simulink/Logic and Bit Operations/Compare To Constant  relop=>=  const=quadModel.minThr  OutDataTypeStr=uint8
  Product : Product
  Sum1 : Sum  Inputs=++|
  Out5 : Outport  VectorParamsAs1DForOutWhenUnconnected=off
  wires:
  Constant/1 -> Sum1/1
  Sum1/1 -> Product/1
  Gain/1 -> Sum1/2
  In5/1 -> Minimum Throttle Cutoff/1, Gain/1
  Product/1 -> Out5/1
  Minimum Throttle Cutoff/1 -> Product/2
